simulink model "AV_homo_traffic"  (R2020b)
settings: Solver=FixedStepAuto  StartTime=0.0  StopTime=3600  FixedStep=0.02  RelTol=1e-3
model workspace (MAT data in the model file):
  P_a_x = [-10 0 10]
  P_a_y = [-12.8017053517 0 14.85382]
  P_v_x = [-100 0 100]
  P_v_y = [-10.4028259584 0 12.0704]
  Range_Sensor = 250
  Set_Speeds = [50 100 150]
  a_max_x = [0 5 20 50]
  a_max_y = [7.811082 7.811082 3.905541 3.905541]
  a_min_x = [-1 0 0.0001 5 20 50]
  a_min_y = [0 0 -5 -5 -3.5 -3.5]
  cycle_dovt = [0 0 0 0 0 0 0 0 0 0 0 0 ... (21081 elements, 1x21081)]
  cycle_t = [0 0.05 0.1 0.15 0.2 0.25 0.3 0.35 0.4 0.45 0.5 0.55 ... (21361 elements, 1x21361)]
  cycle_type = [3 3 3 3 3 3 3 3 3 3 3 3 ... (21081 elements, 1x21081)]
  cycle_v = [0 0 0 0 0 0 0 0 0 0 0 0 ... (21361 elements, 1x21361)]
  cycle_x = [0 0 0 0 0 0 0 0 0 0 0 0 ... (21361 elements, 1x21361)]
  cycle_xx = [0 9.74820143885e-05 0.000573141486811 0.0017757793765 0.00401894484412 0.0075809352518 0.0127047961631 0.0195983213429 0.0284340527578 0.0393492805755 0.0524460431655 0.0677911270983 ... (21081 elements, 1x21081)]
  d0 = 2
  j_min_x = [0 5 20 50]
  j_min_y = [-8.608244 -8.608244 -4.304122 -4.304122]
  ovt_tol = 11.163335
  set_speeds = [50 100 137.38231]
  t_delta_traf = 10
  t_sensor = 0.2
  t_set = 0.651096
libraries: simulink x6
(part 2 of 2)

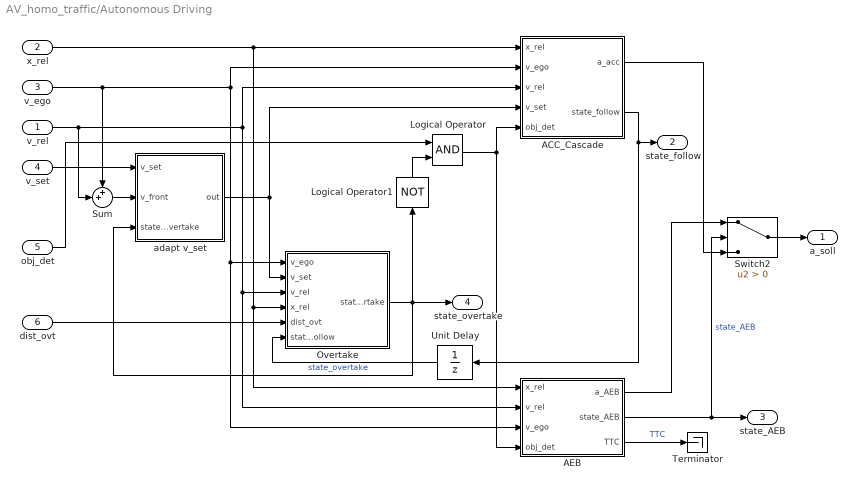
== system AV_homo_traffic/Autonomous Driving ==
  v_rel : Inport  Unit=m/s
  x_rel : Inport  Port=2  Unit=m
  v_ego : Inport  Port=3  Unit=m/s
  v_set : Inport  Port=4  Unit=km/h
  obj_det : Inport  Port=5
  dist_ovt : Inport  Port=6
  ACC_Cascade : Subsystem
  AEB : Subsystem
  Logical Operator : Logic  AllPortsSameDT=off  OutDataTypeStr=boolean
  Logical Operator1 : Logic  Operator=NOT  AllPortsSameDT=off  OutDataTypeStr=boolean
  Overtake : Subsystem
  Sum : Sum  Inputs=++|
  Switch2 : Switch  Criteria=u2 > Threshold
  Terminator : Terminator
  Unit Delay : UnitDelay  SampleTime=-1  HasFrameUpgradeWarning=on
  adapt v_set : Subsystem
  a_soll : Outport  Unit=m/s^2
  state_follow : Outport  Port=2  OutDataTypeStr=boolean
  state_AEB : Outport  Port=3  OutDataTypeStr=boolean
  state_overtake : Outport  Port=4  OutDataTypeStr=boolean
  wires:
  x_rel/1 -> AEB/1(x_rel), Overtake/4(x_rel), ACC_Cascade/1(x_rel)
  v_rel/1 -> AEB/2(v_rel), Overtake/3(v_rel), ACC_Cascade/3(v_rel), Sum/2
  obj_det/1 -> Logical Operator/1
  v_ego/1 -> AEB/3(v_ego), Overtake/1(v_ego), ACC_Cascade/2(v_ego), Sum/1
  Switch2/1 -> a_soll/1
  AEB/3(TTC) -> Terminator/1  "TTC"
  AEB/1(a_AEB) -> Switch2/1
  AEB/2(state_AEB) -> state_AEB/1, Switch2/2  "state_AEB"
  ACC_Cascade/1(a_acc) -> Switch2/3
  ACC_Cascade/2(state_follow) -> Unit Delay/1, state_follow/1
  Logical Operator/1 -> ACC_Cascade/5(obj_det), AEB/4(obj_det)
  Overtake/1(state_overtake) -> state_overtake/1, adapt v_set/3(state_overtake), Logical Operator1/1  "state_overtake"
  dist_ovt/1 -> Overtake/5(dist_ovt)
  Logical Operator1/1 -> Logical Operator/2
  adapt v_set/1(out) -> ACC_Cascade/4(v_set), Overtake/2(v_set)
  Unit Delay/1 -> Overtake/6(state_follow)
  v_set/1 -> adapt v_set/1(v_set)
  Sum/1 -> adapt v_set/2(v_front)

== system AV_homo_traffic/Ego-Vehicle ==
  a_soll : Inport  Unit=m/s^2
  Integrator : Integrator
  Integrator1 : Integrator
  Powertrain : Subsystem
  Saturation1 : Saturate  UpperLimit=100  LowerLimit=0
  a_ego : Outport  Unit=m/s^2
  v_ego : Outport  Port=2
  x_ego : Outport  Port=3
  wires:
  Integrator1/1 -> x_ego/1
  Saturation1/1 -> v_ego/1, Integrator1/1, Powertrain/2(v_ego)
  a_soll/1 -> Powertrain/1(a_soll)
  Integrator/1 -> Saturation1/1
  Powertrain/1(a_ist) -> a_ego/1, Integrator/1

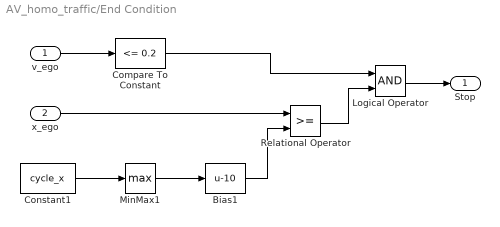
== system AV_homo_traffic/End Condition ==
  v_ego : Inport
  x_ego : Inport  Port=2
  Bias1 : Bias  Bias=-10
  Compare To Constant : simulink/Logic and Bit Operations/Compare To Constant  relop=<=  const=0.2  OutDataTypeStr=boolean
  Constant1 : Constant  Value=cycle_x
  Logical Operator : Logic  AllPortsSameDT=off  OutDataTypeStr=boolean
  MinMax1 : MinMax  Function=max
  Relational Operator : RelationalOperator  OutDataTypeStr=boolean  RndMeth=Simplest
  Stop : Outport
  wires:
  v_ego/1 -> Compare To Constant/1
  Constant1/1 -> MinMax1/1
  MinMax1/1 -> Bias1/1
  x_ego/1 -> Relational Operator/1
  Bias1/1 -> Relational Operator/2
  Relational Operator/1 -> Logical Operator/2
  Compare To Constant/1 -> Logical Operator/1
  Logical Operator/1 -> Stop/1

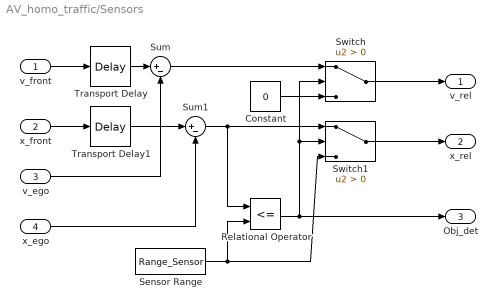
== system AV_homo_traffic/Sensors ==
  v_front : Inport  Unit=m/s
  x_front : Inport  Port=2  Unit=m
  v_ego : Inport  Port=3  Unit=m/s
  x_ego : Inport  Port=4  Unit=m
  Constant : Constant  Value=0
  Relational Operator : RelationalOperator  Operator=<=  OutDataTypeStr=boolean  RndMeth=Simplest
  Sensor Range : Constant  Value=Range_Sensor
  Sum : Sum  Inputs=|+-
  Sum1 : Sum  Inputs=|+-
  Switch : Switch  Criteria=u2 > Threshold
  Switch1 : Switch  Criteria=u2 > Threshold
  Transport Delay : TransportDelay  DelayTime=t_sensor
  Transport Delay1 : TransportDelay  DelayTime=t_sensor
  v_rel : Outport
  x_rel : Outport  Port=2
  Obj_det : Outport  Port=3  OutDataTypeStr=boolean
  wires:
  v_ego/1 -> Sum/2
  x_front/1 -> Transport Delay1/1
  x_ego/1 -> Sum1/2
  Sum1/1 -> Switch1/1, Relational Operator/1
  Relational Operator/1 -> Switch1/2, Switch/2, Obj_det/1
  Switch/1 -> v_rel/1
  Switch1/1 -> x_rel/1
  Sum/1 -> Switch/1
  Constant/1 -> Switch/3
  Sensor Range/1 -> Relational Operator/2, Switch1/3
  Transport Delay/1 -> Sum/1
  v_front/1 -> Transport Delay/1
  Transport Delay1/1 -> Sum1/1

== system AV_homo_traffic/Set_Speed ==
  Road_Type : Inport
  Constant : Constant  Value=set_speeds
  Index Vector : MultiPortSwitch  Inputs=1
  Set_Speed : Outport  Unit=km/h
  wires:
  Road_Type/1 -> Index Vector/1
  Index Vector/1 -> Set_Speed/1
  Constant/1 -> Index Vector/2

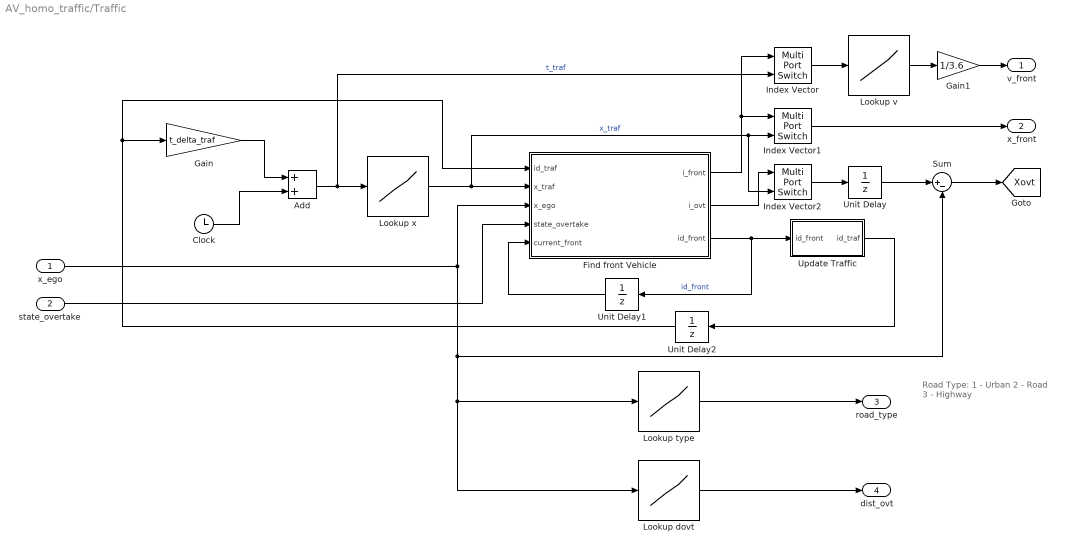
== system AV_homo_traffic/Traffic ==
  note: Road Type:
      | 1 - Urban
      | 2 - Road
      | 3 - Highway
  x_ego : Inport  Unit=m
  state_overtake : Inport  Port=2
  Add : Sum
  Clock : Clock
  Find front Vehicle : MATLAB Function  TreatAsAtomicUnit=on
  Gain : Gain  Gain=t_delta_traf
  Gain1 : Gain  Gain=1/3.6
  Index Vector : MultiPortSwitch  Inputs=1
  Index Vector1 : MultiPortSwitch  Inputs=1
  Index Vector2 : MultiPortSwitch  Inputs=1
  Lookup dovt : Lookup_n-D  NumberOfTableDimensions=1  BreakpointsForDimension1=cycle_xx  Table=cycle_dovt  InterpMethod=Flat  InternalRulePriority=Speed  RndMeth=Simplest  InputSameDT=on
  Lookup type : Lookup_n-D  NumberOfTableDimensions=1  BreakpointsForDimension1=cycle_xx  Table=cycle_type  InterpMethod=Flat  InternalRulePriority=Speed  RndMeth=Simplest  InputSameDT=on
  Lookup v : Lookup_n-D  NumberOfTableDimensions=1  BreakpointsForDimension1=cycle_t  Table=cycle_v  ExtrapMethod=Clip  UseLastTableValue=on  InternalRulePriority=Speed  RndMeth=Simplest  InputSameDT=on
  Lookup x : Lookup_n-D  NumberOfTableDimensions=1  BreakpointsForDimension1=cycle_t  Table=cycle_x  ExtrapMethod=Clip  UseLastTableValue=on  InternalRulePriority=Speed  RndMeth=Simplest  InputSameDT=on
  Sum : Sum  Inputs=|+-
  Unit Delay : UnitDelay  SampleTime=-1  HasFrameUpgradeWarning=on
  Unit Delay1 : UnitDelay  SampleTime=-1  HasFrameUpgradeWarning=on
  Unit Delay2 : UnitDelay  InitialCondition=[-1,0,1]  SampleTime=-1  HasFrameUpgradeWarning=on
  Update Traffic : Subsystem
  v_front : Outport  Unit=m/s
  x_front : Outport  Port=2  Unit=m
  road_type : Outport  Port=3
  dist_ovt : Outport  Port=4  Unit=m
  tag scope: Xovt=global
  wires:
  Add/1 -> Index Vector/2, Lookup x/1  "t_traf"
  Clock/1 -> Add/2
  Gain/1 -> Add/1
  Lookup x/1 -> Find front Vehicle/2(x_traf), Index Vector2/2, Index Vector1/2  "x_traf"
  x_ego/1 -> Sum/2, Lookup dovt/1, Lookup type/1, Find front Vehicle/3(x_ego)
  state_overtake/1 -> Find front Vehicle/4(state_overtake)
  Find front Vehicle/3(id_front) -> Update Traffic/1(id_front), Unit Delay1/1  "id_front"
  Index Vector/1 -> Lookup v/1
  Lookup v/1 -> Gain1/1
  Index Vector1/1 -> x_front/1
  Unit Delay1/1 -> Find front Vehicle/5(current_front)
  Unit Delay2/1 -> Find front Vehicle/1(id_traf), Gain/1
  Lookup type/1 -> road_type/1
  Lookup dovt/1 -> dist_ovt/1
  Gain1/1 -> v_front/1
  Find front Vehicle/1(i_front) -> Index Vector/1, Index Vector1/1
  Update Traffic/1(id_traf) -> Unit Delay2/1
  Find front Vehicle/2(i_ovt) -> Index Vector2/1
  Index Vector2/1 -> Unit Delay/1
  Sum/1 -> [Xovt]
  Unit Delay/1 -> Sum/1

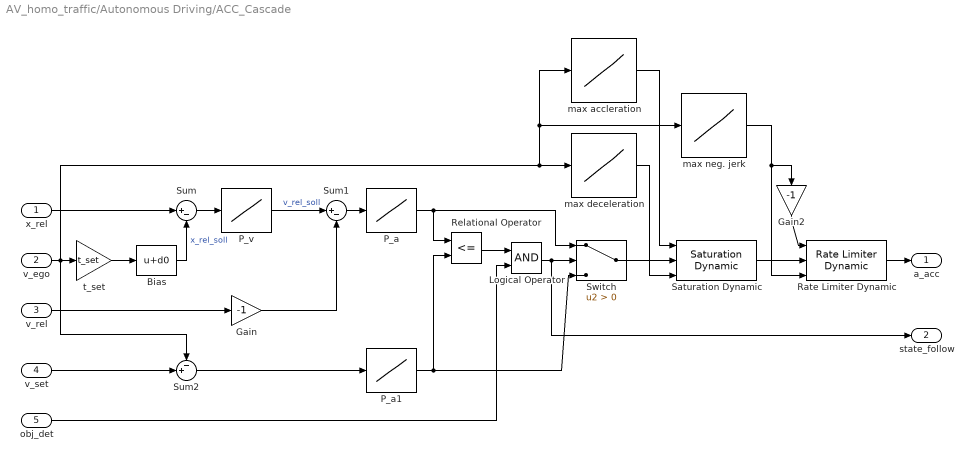
== system AV_homo_traffic/Autonomous Driving/ACC_Cascade ==
  x_rel : Inport  Unit=m
  v_ego : Inport  Port=2  Unit=m/s
  v_rel : Inport  Port=3  Unit=m/s
  v_set : Inport  Port=4  Unit=m/s
  obj_det : Inport  Port=5
  Bias : Bias  Bias=d0
  Gain : Gain  Gain=-1
  Gain2 : Gain  Gain=-1
  Logical Operator : Logic  AllPortsSameDT=off  OutDataTypeStr=boolean
  P_a : Lookup_n-D  NumberOfTableDimensions=1  BreakpointsForDimension1=P_a_x  Table=P_a_y  InternalRulePriority=Speed  RndMeth=Simplest  InputSameDT=on
  P_a1 : Lookup_n-D  NumberOfTableDimensions=1  BreakpointsForDimension1=P_a_x  Table=P_a_y  InternalRulePriority=Speed  RndMeth=Simplest  InputSameDT=on
  P_v : Lookup_n-D  NumberOfTableDimensions=1  BreakpointsForDimension1=P_v_x  Table=P_v_y  InternalRulePriority=Speed  RndMeth=Simplest  InputSameDT=on
  Rate Limiter Dynamic : simulink/Discontinuities/Rate Limiter Dynamic
  Relational Operator : RelationalOperator  Operator=<=  OutDataTypeStr=boolean  RndMeth=Simplest
  Saturation Dynamic : simulink/Discontinuities/Saturation Dynamic  OutMin=[]  OutMax=[]  OutDataTypeStr=Inherit: Same as second input  OutDataType=fixdt(1, 16)  OutScaling=2^-10  DoSatur=off
  Sum : Sum  Inputs=|+-
  Sum1 : Sum  Inputs=|+-
  Sum2 : Sum  Inputs=-+|
  Switch : Switch  Criteria=u2 > Threshold
  max accleration : Lookup_n-D  NumberOfTableDimensions=1  BreakpointsForDimension1=a_max_x  Table=a_max_y  InternalRulePriority=Speed  RndMeth=Simplest  InputSameDT=on
  max deceleration : Lookup_n-D  NumberOfTableDimensions=1  BreakpointsForDimension1=a_min_x  Table=a_min_y  InternalRulePriority=Speed  RndMeth=Simplest  InputSameDT=on
  max neg. jerk : Lookup_n-D  NumberOfTableDimensions=1  BreakpointsForDimension1=j_min_x  Table=j_min_y  InternalRulePriority=Speed  RndMeth=Simplest  InputSameDT=on
  t_set : Gain  Gain=t_set
  a_acc : Outport
  state_follow : Outport  Port=2  OutDataTypeStr=boolean
  wires:
  Gain2/1 -> Rate Limiter Dynamic/1
  P_a1/1 -> Switch/3, Relational Operator/2
  max deceleration/1 -> Saturation Dynamic/3
  x_rel/1 -> Sum/1
  Rate Limiter Dynamic/1 -> a_acc/1
  max neg. jerk/1 -> Gain2/1, Rate Limiter Dynamic/3
  max accleration/1 -> Saturation Dynamic/1
  Sum1/1 -> P_a/1
  v_set/1 -> Sum2/2
  v_ego/1 -> t_set/1, Sum2/1, max accleration/1, max neg. jerk/1, max deceleration/1
  Relational Operator/1 -> Logical Operator/1
  Saturation Dynamic/1 -> Rate Limiter Dynamic/2
  Switch/1 -> Saturation Dynamic/2
  P_a/1 -> Switch/1, Relational Operator/1
  t_set/1 -> Bias/1
  obj_det/1 -> Logical Operator/2
  Sum2/1 -> P_a1/1
  Gain/1 -> Sum1/2
  Bias/1 -> Sum/2  "x_rel_soll"
  v_rel/1 -> Gain/1
  Logical Operator/1 -> state_follow/1, Switch/2
  Sum/1 -> P_v/1
  P_v/1 -> Sum1/1  "v_rel_soll"

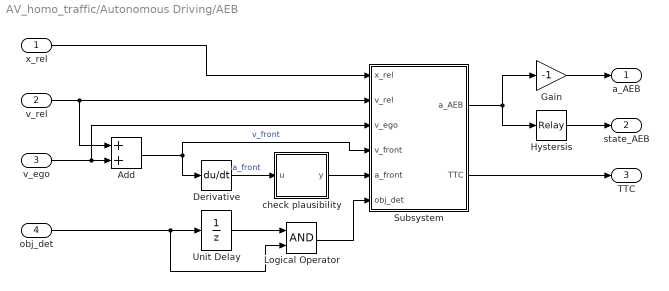
== system AV_homo_traffic/Autonomous Driving/AEB ==
  x_rel : Inport
  v_rel : Inport  Port=2
  v_ego : Inport  Port=3
  obj_det : Inport  Port=4
  Add : Sum
  Derivative : Derivative
  Gain : Gain  Gain=-1
  Hystersis : Relay  OnSwitchValue=5  OffSwitchValue=1  OutDataTypeStr=Inherit: Inherit via back propagation
  Logical Operator : Logic  AllPortsSameDT=off  OutDataTypeStr=boolean
  Subsystem : Subsystem
  Unit Delay : UnitDelay  SampleTime=-1  HasFrameUpgradeWarning=on
  check plausibility : MATLAB Function  TreatAsAtomicUnit=on
  a_AEB : Outport
  state_AEB : Outport  Port=2  OutDataTypeStr=boolean
  TTC : Outport  Port=3
  wires:
  v_rel/1 -> Add/1, Subsystem/2(v_rel)
  v_ego/1 -> Subsystem/3(v_ego), Add/2
  Add/1 -> Subsystem/4(v_front), Derivative/1  "v_front"
  Hystersis/1 -> state_AEB/1
  obj_det/1 -> Logical Operator/2, Unit Delay/1
  Unit Delay/1 -> Logical Operator/1
  Subsystem/1(a_AEB) -> Gain/1, Hystersis/1
  x_rel/1 -> Subsystem/1(x_rel)
  Gain/1 -> a_AEB/1
  Derivative/1 -> check plausibility/1(u)  "a_front"
  Logical Operator/1 -> Subsystem/6(obj_det)
  check plausibility/1(y) -> Subsystem/5(a_front)
  Subsystem/2(TTC) -> TTC/1

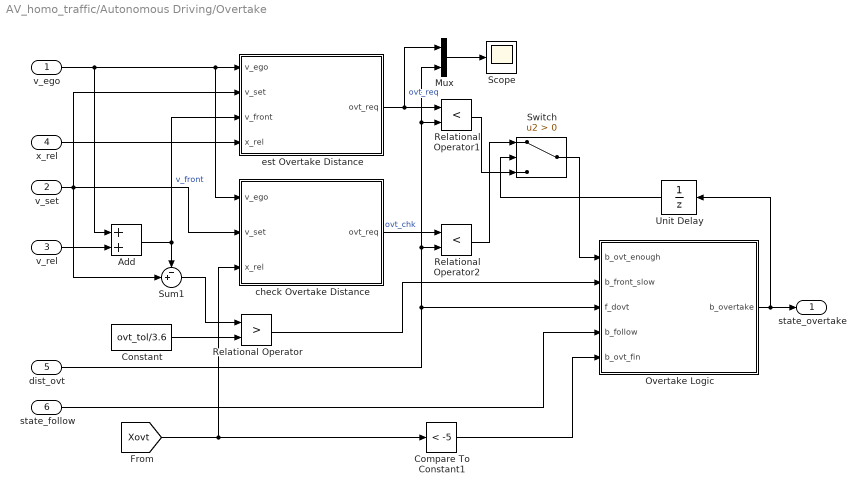
== system AV_homo_traffic/Autonomous Driving/Overtake ==
  v_ego : Inport  Unit=m/s
  v_set : Inport  Port=2  Unit=m/s
  v_rel : Inport  Port=3  Unit=m/s
  x_rel : Inport  Port=4  Unit=m
  dist_ovt : Inport  Port=5  Unit=m
  state_follow : Inport  Port=6
  Add : Sum
  Compare To Constant1 : simulink/Logic and Bit Operations/Compare To Constant  relop=<  const=-5  OutDataTypeStr=boolean
  Constant : Constant  Value=ovt_tol/3.6
  Mux : Mux  Inputs=2
  Overtake Logic : Stateflow chart  TreatAsAtomicUnit=on
  Relational Operator : RelationalOperator  Operator=>  OutDataTypeStr=boolean  RndMeth=Simplest
  Relational Operator1 : RelationalOperator  Operator=<  OutDataTypeStr=boolean  RndMeth=Simplest
  Relational Operator2 : RelationalOperator  Operator=<  OutDataTypeStr=boolean  RndMeth=Simplest
  Scope : Scope
  Sum1 : Sum  Inputs=-+|
  Switch : Switch  Criteria=u2 > Threshold
  Unit Delay : UnitDelay  SampleTime=-1  HasFrameUpgradeWarning=on
  check Overtake Distance : Subsystem
  est Overtake Distance : Subsystem
  state_overtake : Outport  OutDataTypeStr=boolean
  wires:
  v_rel/1 -> Add/2
  Constant/1 -> Relational Operator/2
  Relational Operator/1 -> Overtake Logic/2(b_front_slow)
  Add/1 -> est Overtake Distance/3(v_front), Sum1/1  "v_front"
  dist_ovt/1 -> Relational Operator2/2, Relational Operator1/2, Mux/2, Overtake Logic/3(f_dovt)
  Overtake Logic/1(b_overtake) -> state_overtake/1, Unit Delay/1
  Mux/1 -> Scope/1
  Sum1/1 -> Relational Operator/1
  [Xovt] -> Compare To Constant1/1, check Overtake Distance/3(x_rel)
  Compare To Constant1/1 -> Overtake Logic/5(b_ovt_fin)
  state_follow/1 -> Overtake Logic/4(b_follow)
  check Overtake Distance/1(ovt_req) -> Relational Operator2/1  "ovt_chk"
  Switch/1 -> Overtake Logic/1(b_ovt_enough)
  Relational Operator2/1 -> Switch/1
  v_ego/1 -> check Overtake Distance/1(v_ego), est Overtake Distance/1(v_ego), Add/1
  est Overtake Distance/1(ovt_req) -> Relational Operator1/1, Mux/1  "ovt_req"
  x_rel/1 -> est Overtake Distance/4(x_rel)
  Relational Operator1/1 -> Switch/3
  Unit Delay/1 -> Switch/2
  v_set/1 -> est Overtake Distance/2(v_set), check Overtake Distance/2(v_set), Sum1/2

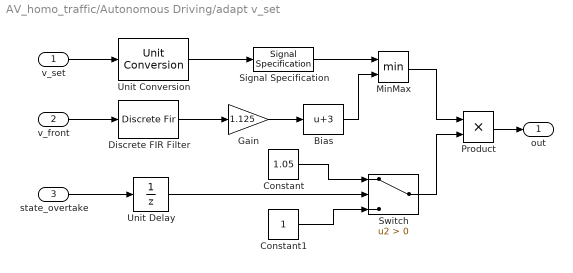
== system AV_homo_traffic/Autonomous Driving/adapt v_set ==
  v_set : Inport  Unit=km/h
  v_front : Inport  Port=2
  state_overtake : Inport  Port=3
  Bias : Bias  Bias=3
  Constant : Constant  Value=1.05
  Constant1 : Constant
  Discrete FIR Filter : DiscreteFir  Coefficients=ones(1,40)/40
  Gain : Gain  Gain=1.125
  MinMax : MinMax  Inputs=2
  Product : Product
  Signal Specification : SignalSpecification  Unit=m/s
  Switch : Switch  Criteria=u2 > Threshold
  Unit Conversion : UnitConversion  OutputType=Inherit: Inherit via back propagation
  Unit Delay : UnitDelay  SampleTime=-1  HasFrameUpgradeWarning=on
  out : Outport  Unit=m/s
  wires:
  v_front/1 -> Discrete FIR Filter/1
  Gain/1 -> Bias/1
  v_set/1 -> Unit Conversion/1
  Bias/1 -> MinMax/2
  Discrete FIR Filter/1 -> Gain/1
  Unit Conversion/1 -> Signal Specification/1
  Signal Specification/1 -> MinMax/1
  state_overtake/1 -> Unit Delay/1
  Constant1/1 -> Switch/3
  Constant/1 -> Switch/1
  MinMax/1 -> Product/1
  Switch/1 -> Product/2
  Product/1 -> out/1
  Unit Delay/1 -> Switch/2

== system AV_homo_traffic/Ego-Vehicle/Powertrain ==
  a_soll : Inport
  v_ego : Inport  Port=2
  Constant : Constant  Value=-8
  Constant1 : Constant  Value=5
  Low speed : Subsystem
  PT1 : TransferFcn  Denominator=[0.2 1]
  Saturation Dynamic : simulink/Discontinuities/Saturation Dynamic  OutMin=[]  OutMax=[]  OutDataTypeStr=Inherit: Same as second input  OutDataType=fixdt(1, 16)  OutScaling=2^-10  DoSatur=off
  a_ist : Outport
  wires:
  a_soll/1 -> Saturation Dynamic/2
  Constant/1 -> Saturation Dynamic/3
  Constant1/1 -> Saturation Dynamic/1
  v_ego/1 -> Low speed/2(v)
  Saturation Dynamic/1 -> Low speed/1(a)
  Low speed/1(a_out) -> PT1/1
  PT1/1 -> a_ist/1

== system AV_homo_traffic/Traffic/Update Traffic ==
  id_front : Inport
  Add : Sum
  Constant : Constant  Value=[-1,0,1]
  Update Traffic : MATLAB Function  Commented=on  TreatAsAtomicUnit=on
  id_traf : Outport
  wires:
  Add/1 -> id_traf/1
  id_front/1 -> Add/2
  Constant/1 -> Add/1

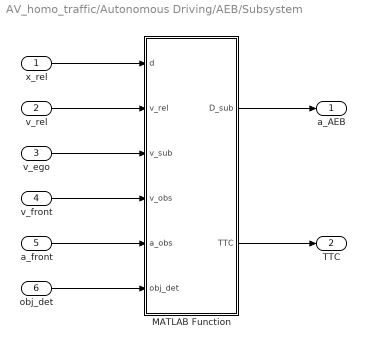
== system AV_homo_traffic/Autonomous Driving/AEB/Subsystem ==
  x_rel : Inport
  v_rel : Inport  Port=2
  v_ego : Inport  Port=3
  v_front : Inport  Port=4
  a_front : Inport  Port=5
  obj_det : Inport  Port=6
  MATLAB Function : MATLAB Function  TreatAsAtomicUnit=on
  a_AEB : Outport
  TTC : Outport  Port=2
  wires:
  x_rel/1 -> MATLAB Function/1(d)
  v_rel/1 -> MATLAB Function/2(v_rel)
  v_ego/1 -> MATLAB Function/3(v_sub)
  v_front/1 -> MATLAB Function/4(v_obs)
  a_front/1 -> MATLAB Function/5(a_obs)
  MATLAB Function/1(D_sub) -> a_AEB/1
  obj_det/1 -> MATLAB Function/6(obj_det)
  MATLAB Function/2(TTC) -> TTC/1

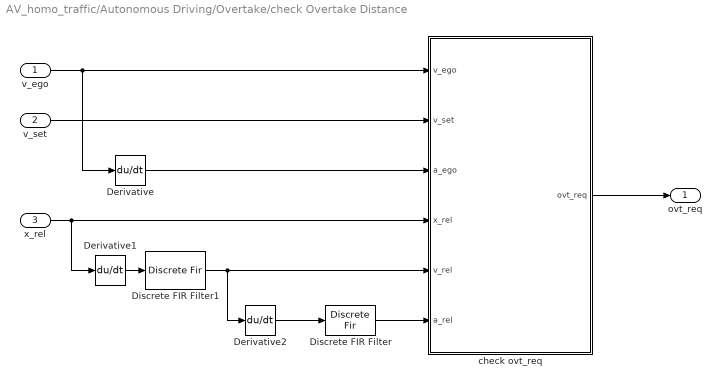
== system AV_homo_traffic/Autonomous Driving/Overtake/check Overtake Distance ==
  v_ego : Inport
  v_set : Inport  Port=2
  x_rel : Inport  Port=3
  Derivative : Derivative
  Derivative1 : Derivative
  Derivative2 : Derivative
  Discrete FIR Filter : DiscreteFir  Coefficients=[10:-1:1]/sum([1:10])
  Discrete FIR Filter1 : DiscreteFir  Coefficients=[5,4,3,2,1]/15
  check ovt_req : MATLAB Function  TreatAsAtomicUnit=on
  ovt_req : Outport
  wires:
  x_rel/1 -> Derivative1/1, check ovt_req/4(x_rel)
  v_set/1 -> check ovt_req/2(v_set)
  v_ego/1 -> Derivative/1, check ovt_req/1(v_ego)
  check ovt_req/1(ovt_req) -> ovt_req/1
  Derivative/1 -> check ovt_req/3(a_ego)
  Discrete FIR Filter1/1 -> Derivative2/1, check ovt_req/5(v_rel)
  Derivative2/1 -> Discrete FIR Filter/1
  Discrete FIR Filter/1 -> check ovt_req/6(a_rel)
  Derivative1/1 -> Discrete FIR Filter1/1

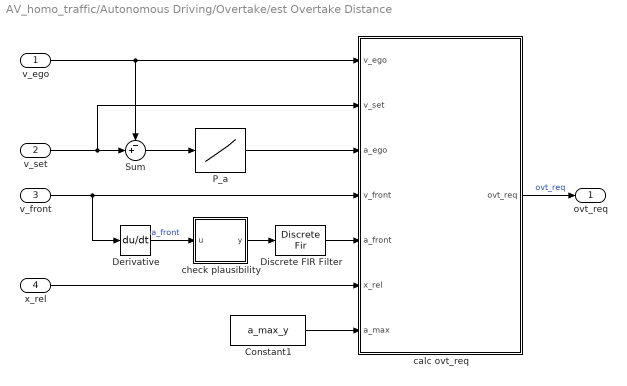
== system AV_homo_traffic/Autonomous Driving/Overtake/est Overtake Distance ==
  v_ego : Inport
  v_set : Inport  Port=2
  v_front : Inport  Port=3
  x_rel : Inport  Port=4
  Constant1 : Constant  Value=a_max_y
  Derivative : Derivative
  Discrete FIR Filter : DiscreteFir  Coefficients=[5,4,3,2,1]/15
  P_a : Lookup_n-D  NumberOfTableDimensions=1  BreakpointsForDimension1=P_a_x  Table=P_a_y  InternalRulePriority=Speed  RndMeth=Simplest  InputSameDT=on
  Sum : Sum  Inputs=-+|
  calc ovt_req : MATLAB Function  TreatAsAtomicUnit=on
  check plausibility : MATLAB Function  TreatAsAtomicUnit=on
  ovt_req : Outport
  wires:
  P_a/1 -> calc ovt_req/3(a_ego)
  calc ovt_req/1(ovt_req) -> ovt_req/1  "ovt_req"
  v_front/1 -> Derivative/1, calc ovt_req/4(v_front)
  v_set/1 -> calc ovt_req/2(v_set), Sum/2
  Sum/1 -> P_a/1
  Derivative/1 -> check plausibility/1(u)  "a_front"
  Constant1/1 -> calc ovt_req/7(a_max)
  check plausibility/1(y) -> Discrete FIR Filter/1
  v_ego/1 -> calc ovt_req/1(v_ego), Sum/1
  x_rel/1 -> calc ovt_req/6(x_rel)
  Discrete FIR Filter/1 -> calc ovt_req/5(a_front)

== system AV_homo_traffic/Ego-Vehicle/Powertrain/Low speed ==
  a : Inport
  v : Inport  Port=2
  MATLAB Function : MATLAB Function  TreatAsAtomicUnit=on
  a_out : Outport
  wires:
  a/1 -> MATLAB Function/1("a ")
  v/1 -> MATLAB Function/2(v)
  MATLAB Function/1(a) -> a_out/1

== matlab function AV_homo_traffic/Autonomous Driving/Overtake/est Overtake Distance/calc ovt_req ==
  data: v_ego input; ovt_req output; v_set input; a_ego input; v_front input; a_front input; x_rel input; a_max input
function ovt_req = calc_ovt_dist(v_ego, v_set, a_ego, v_front, a_front, x_rel, a_max)
    % ovt_req = inf;
    a_ego = min(a_ego, a_max(end));
    x_rel = x_rel + 10; % cut in after overtaken by 5[m], + 5[m] redundancy
    if a_front > a_ego && v_front > v_ego
        ovt_req = inf;
    else
        t_sol = solve_quad1((a_ego - a_front)/2, v_ego - v_front, -x_rel);
        t_acc = max((v_set - v_ego) / a_ego,0);
        if t_sol < t_acc
            ovt_req = v_ego * t_sol + 0.5 * a_ego * t_sol^2;
        else
            x1 = v_ego * t_acc + 0.5 * a_ego * t_acc^2;
            x2 = v_front * t_acc + 0.5 * a_front * t_acc^2;
            v2 = v_front + a_front * t_acc;
            t_sol = solve_quad1( -a_front/2, v_set - v2, -x_rel + x2 - x1);
            ovt_req = x1 + v_set * t_sol;
        end
    end
    if ovt_req > 1000
        ovt_req = inf;
    end
end

function x = solve_quad1(a, b, c)
    % solve quadratic equation
    % return smallest positve real roots
    x = inf;
    if a == 0
        if b ~= 0
            x1 = -c / b;
            if x1 >=0
                x = x1;
            end
        end
    else
        d2 = b^2 - 4 * a * c;
        if d2 >= 0
            d = sqrt(d2);
            x1 = (-b + d) / (2 * a);
            x2 = (-b - d) / (2 * a);
            if x1 >= 0
                x = x1;
            else
                x1 = inf;
            end
            if x2 >= 0 && x2 < x1
                x = x2;
            end
        end
    end
end

== matlab function AV_homo_traffic/Autonomous Driving/Overtake/check Overtake Distance/check ovt_req ==
  data: v_ego input; ovt_req output; v_set input; a_ego input; x_rel input; v_rel input; a_rel input
function ovt_req = check_ovt_dist(v_ego, v_set, a_ego, x_rel, v_rel, a_rel)
    % ovt_req = inf;
    x_rel = x_rel + 5; % cut in after overtaken by 5[m]    
    if a_rel > 0 && v_rel > 0
        ovt_req = inf;
    else
        t_sol = solve_quad1(a_rel/2, v_rel, x_rel);
        t_acc = max((v_set - v_ego) / a_ego,0);
        if t_sol < t_acc
            ovt_req = v_ego * t_sol + 0.5 * a_ego * t_sol^2;
        else
            dx_tacc = v_rel * t_acc + 0.5 * a_rel * t_acc^2;
            v2 = v_rel + a_rel * t_acc;
            t_sol = solve_quad1( (a_rel-a_ego)/2, v2, x_rel + dx_tacc);
            x1 = v_ego * t_acc + 0.5 * a_ego * t_acc^2;
            ovt_req = x1 + v_set * t_sol;
        end
    end
    if ovt_req > 1000
        ovt_req = inf;
    end
end

function x = solve_quad1(a, b, c)
    % solve quadratic equation
    % return smallest positve real roots
    x = inf;
    if a == 0
        if b ~= 0
            x1 = -c / b;
            if x1 >=0
                x = x1;
            end
        end
    else
        d2 = b^2 - 4 * a * c;
        if d2 >= 0
            d = sqrt(d2);
            x1 = (-b + d) / (2 * a);
            x2 = (-b - d) / (2 * a);
            if x1 >= 0
                x = x1;
            else
                x1 = inf;
            end
            if x2 >= 0 && x2 < x1
                x = x2;
            end
        end
    end
end

== matlab function AV_homo_traffic/Ego-Vehicle/Powertrain/Low speed/MATLAB Function ==
  data: a input; a output; v input
function a = lowspeed(a,v)
if v <= 0
    if a < 0.3
        a = 0;
    end
elseif v < 1
    if a < 0
        a = min(a, -0.3);
    elseif a < 0.3
        a = min(a, -0.2);
    end
end

== matlab function AV_homo_traffic/Autonomous Driving/AEB/check plausibility ==
  data: u input; y output
function y = check_a(u)
if abs(u) < 8
    y = u;
else
    y = 0;
end

== matlab function AV_homo_traffic/Autonomous Driving/AEB/Subsystem/MATLAB Function ==
  data: d input; D_sub output; v_rel input; v_sub input; v_obs input; a_obs input; TTC output; obj_det input
function [D_sub,TTC] = fcn(d,v_rel,v_sub,v_obs,a_obs,obj_det)
% Reference: H. Winner, S. Hakuli, F. Lotz, und C. Singer, 
%            Handbuch Fahrerassistenzsysteme: Grundlagen, Komponenten und Systeme für aktive Sicherheit und Komfort, 
%            3rd Aufl. Wiesbaden: Springer Vieweg, 2015.
%            Kapitel 47.6, Seite 899-902
if obj_det && d > 0
    % 1 - not approaching
    if v_rel >= 0
        D_sub = 0;
        TTC = inf;
    else
        v_diff = - v_rel;
        d = max(d - 1, 0.01);
        % 2 - front vehicle not decelerating
        TTC = d / v_diff;
        if a_obs >= 0
            D_sub = v_diff ^2 / (2 * d);
        else
            D_obs = - a_obs;        
            D_sub = 0;
            D_rel = D_obs - D_sub;
            % 3 - front vehicle braking
            %TTC = (sqrt(v_diff ^2 + 2 * D_rel * d) - v_diff)/D_rel;
            if v_obs / D_obs > TTC
                D_sub = D_obs + v_diff ^2 / (2 * d);
            else
                % 4 - front vehicle braking to a stop
                %TTC = (v_sub - sqrt(v_sub ^2 - 2 * D_sub * d - v_obs ^2 * D_sub / D_obs)) / D_sub;
                D_sub = v_sub ^2 /(2 * (d + v_obs ^2 / (2 * D_obs)));
            end
        end
    end
else
    D_sub = 0;
    TTC = inf;
end
D_sub = min(D_sub,10);
if v_sub <= 0
    D_sub = 0;
end

== matlab function AV_homo_traffic/Traffic/Update Traffic/Update Traffic ==
  data: id_front input; id_traf output
function id_traf = update_traffic(id_front)
    % simulate 1 vehicle behind, 2 vehicle in front
    id_traf = [-1, 0, 1] + id_front;
end

== matlab function AV_homo_traffic/Traffic/Find front Vehicle ==
  data: i_front output; i_ovt output; id_traf input; x_traf input; id_front output; x_ego input; state_overtake input boolean; current_front input
function [i_front, i_ovt, id_front] = find_front(id_traf, x_traf, x_ego, state_overtake, current_front)
    % locate current front
    id_front = current_front;
    i_front = find_first(id_traf, id_front);
    % when overtaking, tracking 2 vehicles with i_front & i_ovt
    if state_overtake
        i_ovt = i_front; % the front vehicle being overtaken
        i_front = i_front + 1; % the next vehicle in the front
    else
        % overtake finished
        if x_ego > x_traf(i_front)
            id_front = id_front + 1;
            i_front = i_front + 1;
        % ego-vehicle being overtaken
        elseif x_ego + 20 < x_traf(i_front - 1) % traffic vehicle cut in after 20m
            id_front = id_front - 1;
            i_front = i_front - 1;
        end
        i_ovt = i_front;
    end
end

function i = find_first(v, x)
    for i = 1:length(v)
        if v(i) == x
            break
        end
    end
    if v(i) ~= x
        % warning('Object not find!')
        i = -1;
    end
end

== stateflow chart AV_homo_traffic/Autonomous Driving/Overtake/Overtake Logic ==
  state standby
    b_overtake = false;
  state prepare
  state overtake
    b_overtake = true;
  state aborted
    b_overtake = false;
  state finished
    b_overtake = false;
  (default) -> standby
  aborted -> standby : after(10,sec)
  finished -> standby : after(2,sec)
  prepare -> standby [order 1] : [~(b_ovt_enough & b_front_slow & b_follow & f_dovt>20)]
  standby -> prepare : [b_ovt_enough & b_front_slow & b_follow & f_dovt>20]
  prepare -> overtake [order 2] : after(3,sec)
  overtake -> (junction 25) : after(3,sec)
  (junction 25) -> aborted [order 2] : [~b_ovt_enough]
  (junction 25) -> finished [order 1] : [b_ovt_fin]
  data: b_ovt_enough input boolean; b_front_slow input boolean; b_overtake output boolean; f_dovt input; b_follow input; b_ovt_fin input

== matlab function AV_homo_traffic/Autonomous Driving/Overtake/est Overtake Distance/check plausibility ==
  data: u input; y output
function y = check_a(u)
if abs(u) < 6
    y = u;
else
    y = 0;
end
